simulink model "asyncip_sl_2_sc_console"  (R2021b)
settings: Solver=ode4  StartTime=0.0  StopTime=inf  FixedStep=0.01  MaxStep=0.01  RelTol=1e-3  AbsTol=1e-6
InitFcn:
  | Ns=20;
libraries: opal_lib x3
settings Model: Creator=jwu  LastModifiedBy=NCSLab
settings SolverCC: AutoScaleAbsTol=off  AlgebraicLoopSolver=TrustRegion
settings DataIOCC: ExternalInput=[]  InitialState=[]  SaveFormat=Array  SignalLoggingSaveFormat=ModelDataLogs  SaveOutput=off  SaveTime=off  ReturnWorkspaceOutputs=off  SignalLoggingName=sigsOut
settings OptimizationCC: BooleanDataType=off  OptimizeBlockIOStorage=off  BufferReuse=off  ExpressionFolding=off  LocalBlockOutputs=off  InitFltsAndDblsToZero=on  LifeSpan=inf
settings DebuggingCC: SaveWithParameterizedLinksMsg=none  UnderspecifiedInitializationDetection=Classic  MergeDetectMultiDrivingBlocksExec=none  SignalResolutionControl=TryResolveAllWithWarning  InheritedTsInSrcMsg=none  MultiTaskDSMMsg=warning  MultiTaskCondExecSysMsg=none  FcnCallInpInsideContextMsg=warning  SFUnexpectedBacktrackingDiag=warning  SFNoUnconditionalDefaultTransitionDiag=warning  SFExecutionAtInitializationDiag=none  SFMachineParentedDataDiag=warning  ArithmeticOperatorsInVariantConditions=warning
settings HardwareCC: ProdBitPerPointer=32  ProdBitPerSizeT=32  ProdBitPerPtrDiffT=32  ProdLargestAtomicFloat=None  ProdIntDivRoundTo=Undefined  ProdEndianess=Unspecified  ProdWordSize=32  ProdHWDeviceType=32-bit Generic  TargetUnknown=on
settings ModelReferenceCC: PropagateSignalLabelsOutOfModel=off
settings SFSimCC: SimUseLocalCustomCode=off  CustomCodeUndefinedFunction=UseInterfaceOnly
settings RTWCC: GenCodeOnly=on  RTWUseLocalCustomCode=off
settings CodeAppCC: StateflowObjectComments=on
settings GRTTargetCC: TargetFcnLib=ansi_tfl_tmw.mat  TargetLangStandard=C89/C90 (ANSI)  CombineOutputUpdateFcns=off  GRTInterface=on
settings ConfigComp: CovMetricSettings=dw  CovSaveCumulativeToWorkspaceVar=on  CovSaveSingleToWorkspaceVar=on  CovExternalEMLEnable=off

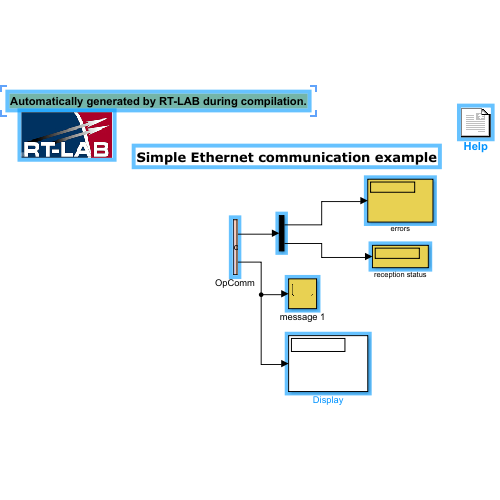
[thumbnail: Simulink's stored preview of the top-level diagram]
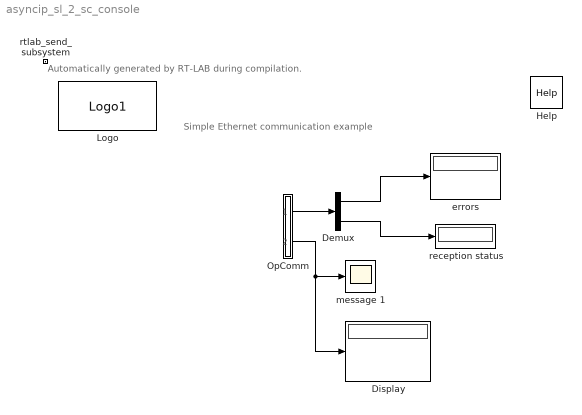
== system asyncip_sl_2_sc_console ==
  note: Automatically generated by RT-LAB during compilation.
  note: Simple Ethernet communication example
  Demux : Demux  Outputs=[2 1]
      settings: DisplayOption=none
  Display : Display
  Help : opal_lib/Help  docfile=../../help/help.simulink.html
  Logo : opal_lib/Logo1  vide=[]
  OpComm : Subsystem
      mask init:
      | opmaskdisplay('maskdisplay_block',gcb,'disp(''OpComm'')');
      mask Display:
      | patch([0 0.5 0.7 0],[1 1 0 0],[0.7 0.75 0.9]);
      | patch([1 0.53 0.73 1],[1 1 0 0],[1 0.8 0.7]);
      | plot([0 0 1 1 0],[0 1 1 0 0]);
      | disp('OpComm')
  errors : Display
  message 1 : Scope
  reception status : Display
  rtlab_send_subsystem : Subsystem  Priority=-100
      mask Display: text(0,0,'');
  wires:
  Demux/2 -> reception status/1
  Demux/1 -> errors/1
  OpComm/1(Out1) -> Demux/1
  OpComm/2(Out2) -> message 1/1, Display/1

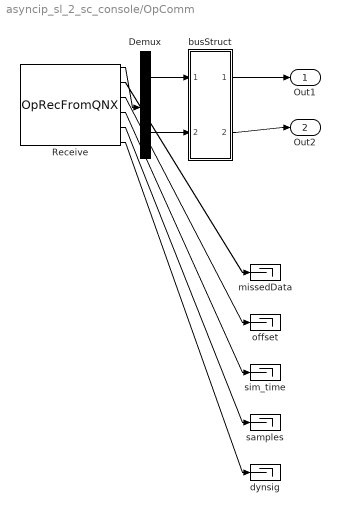
== system asyncip_sl_2_sc_console/OpComm ==
  Demux : Demux  Outputs="[3  3]"
  Receive : opal_lib/Communication/OpRecFromQNX  Node_num=1  Acqu_Group=1  Data_Width=6  Synchronization=on  Interpolation=on  Threshold=1.0  modelname=AsyncIP_sl  sampletime=0.01
  busStruct : Subsystem
  dynsig : Terminator
  missedData : Terminator
  offset : Terminator
  samples : Terminator
  sim_time : Terminator
  Out1 : Outport
  Out2 : Outport  Port=2
  wires:
  Demux/2 -> busStruct/2(In2)
  Demux/1 -> busStruct/1(In1)
  busStruct/2(Out2) -> Out2/1
  busStruct/1(Out1) -> Out1/1
  Receive/1 -> Demux/1
  Receive/6 -> dynsig/1
  Receive/5 -> samples/1
  Receive/4 -> sim_time/1
  Receive/3 -> offset/1
  Receive/2 -> missedData/1

== system asyncip_sl_2_sc_console/rtlab_send_subsystem ==

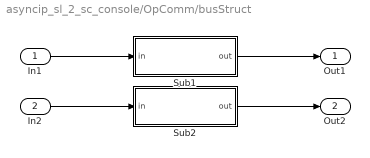
== system asyncip_sl_2_sc_console/OpComm/busStruct ==
  In1 : Inport
  In2 : Inport  Port=2
  Sub1 : Subsystem
  Sub2 : Subsystem
  Out1 : Outport
  Out2 : Outport  Port=2
  wires:
  Sub2/1(out) -> Out2/1
  In2/1 -> Sub2/1(in)
  Sub1/1(out) -> Out1/1
  In1/1 -> Sub1/1(in)

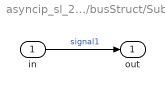
== system asyncip_sl_2_sc_console/OpComm/busStruct/Sub1 ==
  in : Inport
  out : Outport
  wires:
  in/1 -> out/1  "signal1"

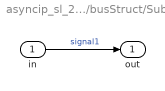
== system asyncip_sl_2_sc_console/OpComm/busStruct/Sub2 ==
  in : Inport
  out : Outport
  wires:
  in/1 -> out/1  "signal1"
